simulink model "model_4_lqg"  (R2022a)
settings: Solver=VariableStepAuto  StartTime=0.0  StopTime=30  RelTol=1e-3
values from neighbouring files (symbols this model uses):
  A = [6, 7, -4, 8; 0, 9, 0, 15; 10, 13, -6, 19; 0, -6, 0, -9]    [task_2.m]
  B = [-8, 0; 4, 0; -6, 0; -2, 0]    [task_2.m]
  C = eye(4)    [task_2.m]
  D = zeros(4, 2)    [task_2.m]
  x0 = [1; -1; 1; -1]    [task_2.m]
undefined symbols (not defined in the file or in its folder): K, L, x_0
settings Model: Creator=vital  LastModifiedBy=Family
settings DebuggingCC: UnconnectedInputMsg=warning  UnconnectedOutputMsg=warning  UnconnectedLineMsg=warning
settings RTWCC: DLArmComputeVersion=19.05

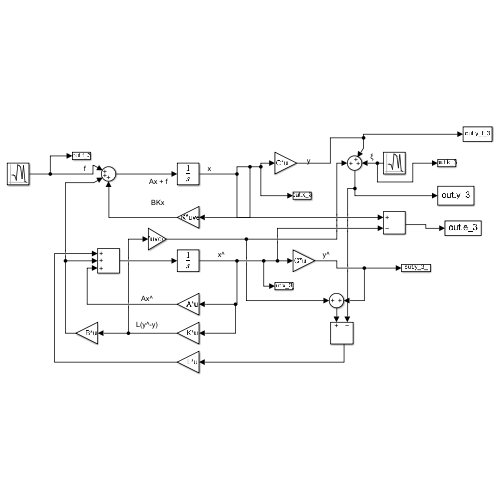
[thumbnail: Simulink's stored preview of the top-level diagram]
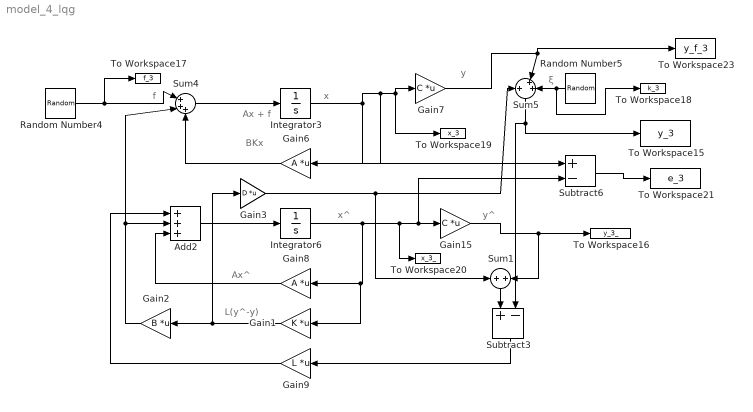
== system model_4_lqg ==
  note: Ax^
  note: BKx
  note: x^
  note: L(y^-y)
  note: x
  note: f
  note: y^
  note: Ax + f
  note: y
  note: ξ
  Add2 : Sum  Inputs=+++
  Gain1 : Gain  Gain=K  Multiplication=Matrix(K*u)
  Gain15 : Gain  Gain=C  Multiplication=Matrix(K*u)
  Gain2 : Gain  Gain=B  Multiplication=Matrix(K*u)
  Gain3 : Gain  Gain=D  Multiplication=Matrix(K*u) (u vector)
  Gain6 : Gain  Gain=A  Multiplication=Matrix(K*u) (u vector)
  Gain7 : Gain  Gain=C  Multiplication=Matrix(K*u)
  Gain8 : Gain  Gain=A  Multiplication=Matrix(K*u)
  Gain9 : Gain  Gain=L  Multiplication=Matrix(K*u)
  Integrator3 : Integrator  InitialCondition=x0
  Integrator6 : Integrator  InitialCondition=x_0
  Random Number4 : RandomNumber  Seed=[13; 14; 15; 16]  SampleTime=0000.1
  Random Number5 : RandomNumber  Seed=[17; 18]  SampleTime=0000.1
  Subtract3 : Sum  Inputs=+-
  Subtract6 : Sum  Inputs=+-
  Sum1 : Sum  Inputs=+|+
  Sum4 : Sum  Inputs=|+++
  Sum5 : Sum  Inputs=+|++
  To Workspace15 : ToWorkspace  VariableName=y_3  SaveFormat=Timeseries  SampleTime=-1
  To Workspace16 : ToWorkspace  VariableName=y_3_  SaveFormat=Timeseries  SampleTime=-1
  To Workspace17 : ToWorkspace  VariableName=f_3  SaveFormat=Timeseries  SampleTime=-1
  To Workspace18 : ToWorkspace  VariableName=k_3  SaveFormat=Timeseries  SampleTime=-1
  To Workspace19 : ToWorkspace  VariableName=x_3  SaveFormat=Timeseries  SampleTime=0.0001
  To Workspace20 : ToWorkspace  VariableName=x_3_  SaveFormat=Timeseries  SampleTime=-1
  To Workspace21 : ToWorkspace  VariableName=e_3  SaveFormat=Timeseries  SampleTime=-1
  To Workspace23 : ToWorkspace  VariableName=y_f_3  SaveFormat=Timeseries  SampleTime=-1
  wires:
  Gain7/1 -> Sum5/2, To Workspace23/1
  Sum4/1 -> Integrator3/1
  Add2/1 -> Integrator6/1
  Gain15/1 -> Sum1/2, To Workspace16/1
  Random Number4/1 -> Sum4/1, To Workspace17/1
  Sum5/1 -> To Workspace15/1, Subtract3/2
  Integrator3/1 -> To Workspace19/1, Gain7/1, Gain6/1, Subtract6/1
  Random Number5/1 -> Sum5/3, To Workspace18/1
  Integrator6/1 -> Gain1/1, Gain8/1, To Workspace20/1, Subtract6/2, Gain15/1
  Subtract6/1 -> To Workspace21/1
  Subtract3/1 -> Gain9/1
  Gain6/1 -> Sum4/3
  Gain8/1 -> Add2/3
  Gain9/1 -> Add2/1
  Gain1/1 -> Gain3/1, Gain2/1
  Gain2/1 -> Sum4/2, Add2/2
  Gain3/1 -> Sum1/1, Sum5/1
  Sum1/1 -> Subtract3/1
